simulink model "comparando_modelo_linear_com_original"  (R2012b)
settings: Solver=ode3  StartTime=0.0  StopTime=1  FixedStep=1e-4  RelTol=1e-6
undefined symbols (not defined in the file or in its folder): tf1
libraries: BLDC x1
settings Model: BufferReuse=off  Creator=Juliano  LastModifiedBy=h3now
settings DataIOCC: LimitDataPoints=off
settings OptimizationCC: OptimizeBlockIOStorage=off  BufferReuse=off  ExpressionFolding=off  LocalBlockOutputs=off

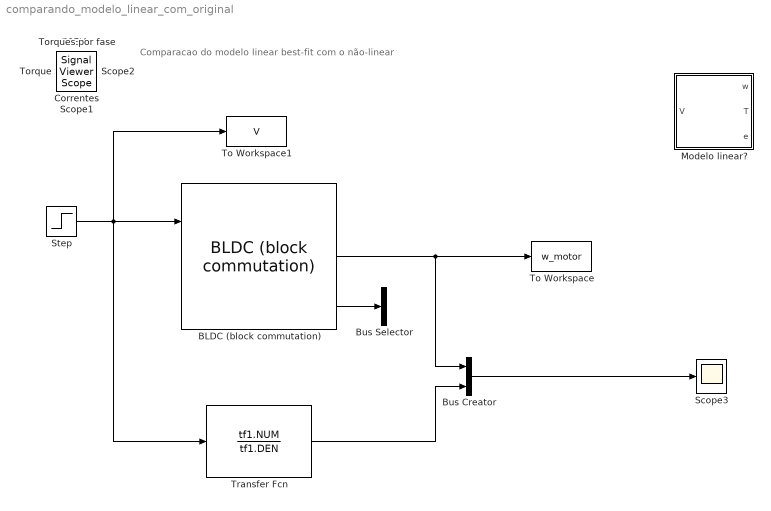
== system comparando_modelo_linear_com_original ==
  note: Comparacao do modelo linear best-fit com o não-linear
  BLDC (block commutation) : BLDC/BLDC (block commutation)  J=1.39e-6  R=10.1/2  L=2.04/2000  P=8  Kt=15.7e-3/1.19  Ke=15.7e-3/1.19  Kd=0
  Bus Creator : BusCreator  Inputs=2
  Bus Selector : BusSelector  OutputSignals=Torque Total,FCEMs
  Modelo linear? : Subsystem  mask{R=10.1/2, L=2.04/2000, Ke=15.7e-3/1.19, Kt=15.7e-3/1.19, J=1.39e-6, Kd=0}
  Scope3 : Scope
      settings: ShowLegends=on
  Step : Step  Time=0  After=6  SampleTime=0
  To Workspace : ToWorkspace  VariableName=w_motor  SampleTime=-1
  To Workspace1 : ToWorkspace  VariableName=V  SampleTime=-1
  Transfer Fcn : TransferFcn  Numerator=tf1.NUM  Denominator=tf1.DEN
  Correntes : SignalViewerScope  IOType=viewer  NumInputPorts=3  ZoomMode=yonly  RefreshTime=0.035000
      settings: YMin=-5~-5~-5  YMax=5~5~5
  FCEMs : SignalViewerScope  IOType=viewer  NumInputPorts=3  ZoomMode=xonly  RefreshTime=0.035000
      settings: YMin=-5~-5~-5  YMax=5~5~5  SaveName=ScopeData2
  Scope1 : SignalViewerScope  IOType=viewer  RefreshTime=0.035000
      settings: SaveName=ScopeData3
  Scope2 : SignalViewerScope  IOType=viewer  RefreshTime=0.035000
      settings: SaveName=ScopeData4
  Torque : SignalViewerScope  IOType=viewer  ZoomMode=xonly  RefreshTime=0.035000
      settings: SaveToWorkspace=on  SaveName=Torque
  Torques por fase : SignalViewerScope  IOType=viewer  NumInputPorts=3  ZoomMode=xonly  RefreshTime=0.035000
      settings: YMin=-5~-5~-5  YMax=5~5~5
  wires:
  Step/1 -> Transfer Fcn/1, To Workspace1/1, BLDC (block commutation)/1
  BLDC (block commutation)/2 -> Bus Creator/1, To Workspace/1
  BLDC (block commutation)/3 -> Bus Selector/1
  Transfer Fcn/1 -> Bus Creator/2
  Bus Creator/1 -> Scope3/1

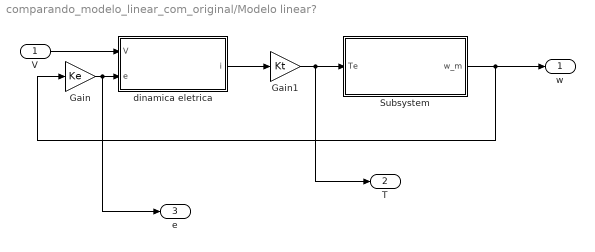
== system comparando_modelo_linear_com_original/Modelo linear? ==
  V : Inport
  Gain : Gain  Gain=Ke
  Gain1 : Gain  Gain=Kt
  Subsystem : Subsystem
  dinamica eletrica : Subsystem
  w : Outport
  T : Outport  Port=2
  e : Outport  Port=3
  wires:
  Gain1/1 -> T/1, Subsystem/1(Te)
  Subsystem/1(w_m) -> w/1, Gain/1
  V/1 -> dinamica eletrica/1(V)
  dinamica eletrica/1(i) -> Gain1/1
  Gain/1 -> e/1, dinamica eletrica/2(e)

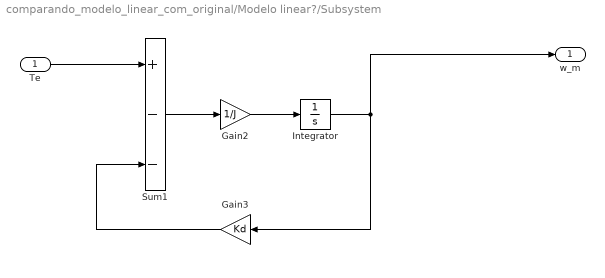
== system comparando_modelo_linear_com_original/Modelo linear?/Subsystem ==
  Te : Inport
  Gain2 : Gain  Gain=1/J
  Gain3 : Gain  Gain=Kd
  Integrator : Integrator
  Sum1 : Sum  Inputs=+--
  w_m : Outport
  wires:
  Gain2/1 -> Integrator/1
  Integrator/1 -> w_m/1, Gain3/1
  Sum1/1 -> Gain2/1
  Gain3/1 -> Sum1/3
  Te/1 -> Sum1/1

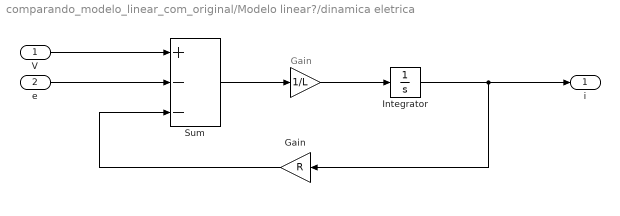
== system comparando_modelo_linear_com_original/Modelo linear?/dinamica eletrica ==
  note: Gain
  V : Inport
  e : Inport  Port=2
  " " : Gain  Gain=1/L
  Gain : Gain  Gain=R
  Integrator : Integrator
  Sum : Sum  Inputs=+--
  i : Outport
  wires:
  V/1 -> Sum/1
  Integrator/1 -> i/1, Gain/1
  Gain/1 -> Sum/3
  e/1 -> Sum/2
  Sum/1 -> " "/1
  " "/1 -> Integrator/1
